simulink library "xbsDSP48_r3"  (Simulink 5.0)
libraries: xbsIndex_r3 x429, xbsDSP48_r3 x2
(part 3 of 8)

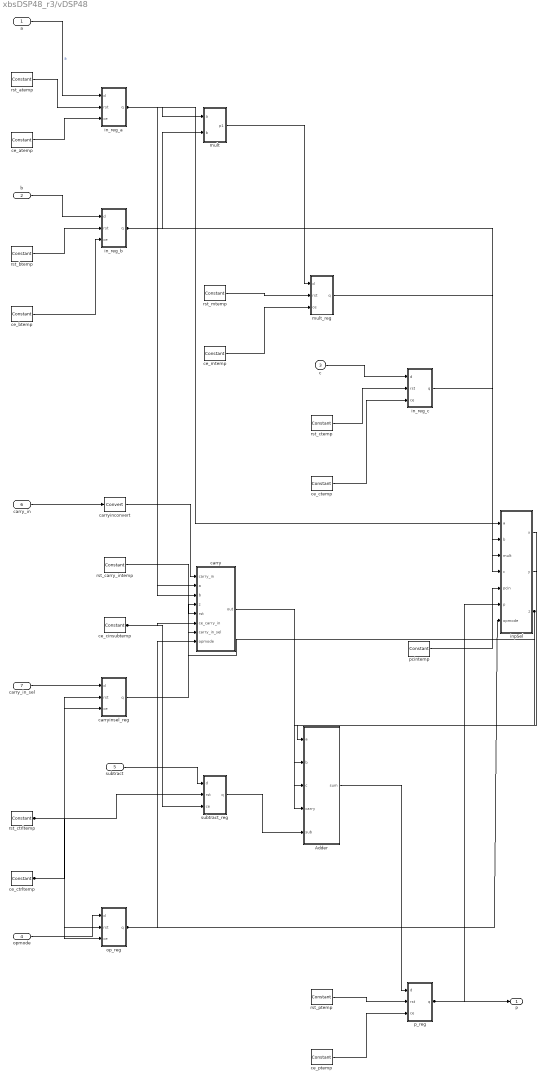
== system xbsDSP48_r3/vDSP48 ==
  a : Inport
  b : Inport  Port=2
  c : Inport  Port=3
  opmode : Inport  Port=4
  subtract : Inport  Port=5
  carry_in : Inport  Port=6
  carry_in_sel : Inport  Port=7
  Adder : Subsystem
  carry : Subsystem
  carryinconvert : xbsIndex_r3/Convert  arith_type=Unsigned  n_bits=1  bin_pt=0  quantization=Truncate  overflow=Wrap  latency=0  explicit_period=off  period=1  dbl_ovrd=off  show_param=off  inserted_by_tool=off  pipeline=off
      settings: xl_area=[0, 0, 0, 0, 0, 0, 0]
  carryinsel_reg : Subsystem  mask{nreg=pipeline_carryinsel, pnreg=1}
      mask prompts: nreg "Number of registers"; pnreg "Previous number of register"
      mask init: same as xbsDSP48_r3/DSP48reg
      mask Display:
      | patch([0 iWidth iWidth 0],[0 0 iHeight iHeight] , bg);
      | patch(logoX,logoY , fg);
      | text(iCx-6,iCy,'z');
      | text(iCx,iCy+4,str);
      | port_label('input',1,'d');
      | port_label('input',2,'rst');
      | port_label('input',3,'ce');
      | port_label('output',1,'q');
      | plot([0 0 iWidth iWidth 0], [0 iHeight iHeight 0 0]);
  ce_atemp : xbsIndex_r3/Constant  const=1  equ=P=C  arith_type=Boolean  n_bits=1  bin_pt=0  opselect=C  inp2=PCIN>>17  opr=+  inp1=P  carry=CIN  iostate=0  explicit_period=on  period=1  dbl_ovrd=off
  ce_btemp : xbsIndex_r3/Constant  const=1  equ=P=C  arith_type=Boolean  n_bits=1  bin_pt=0  opselect=C  inp2=PCIN>>17  opr=+  inp1=P  carry=CIN  iostate=0  explicit_period=on  period=1  dbl_ovrd=off
  ce_cinsubtemp : xbsIndex_r3/Constant  const=1  equ=P=C  arith_type=Boolean  n_bits=1  bin_pt=0  opselect=C  inp2=PCIN>>17  opr=+  inp1=P  carry=CIN  iostate=0  explicit_period=on  period=1  dbl_ovrd=off
  ce_ctemp : xbsIndex_r3/Constant  const=1  equ=P=C  arith_type=Boolean  n_bits=1  bin_pt=0  opselect=C  inp2=PCIN>>17  opr=+  inp1=P  carry=CIN  iostate=0  explicit_period=on  period=1  dbl_ovrd=off
  ce_ctrltemp : xbsIndex_r3/Constant  const=1  equ=P=C  arith_type=Boolean  n_bits=1  bin_pt=0  opselect=C  inp2=PCIN>>17  opr=+  inp1=P  carry=CIN  iostate=0  explicit_period=on  period=1  dbl_ovrd=off
  ce_mtemp : xbsIndex_r3/Constant  const=1  equ=P=C  arith_type=Boolean  n_bits=1  bin_pt=0  opselect=C  inp2=PCIN>>17  opr=+  inp1=P  carry=CIN  iostate=0  explicit_period=on  period=1  dbl_ovrd=off
  ce_ptemp : xbsIndex_r3/Constant  const=1  equ=P=C  arith_type=Boolean  n_bits=1  bin_pt=0  opselect=C  inp2=PCIN>>17  opr=+  inp1=P  carry=CIN  iostate=0  explicit_period=on  period=1  dbl_ovrd=off
  in_reg_a : Subsystem  mask{nreg=pipeline_a-1, pnreg=1}
      mask prompts: nreg "Number of registers"; pnreg "Previous number of register"
      mask init: same as xbsDSP48_r3/DSP48reg
      mask Display:
      | patch([0 iWidth iWidth 0],[0 0 iHeight iHeight] , bg);
      | patch(logoX,logoY , fg);
      | text(iCx-6,iCy,'z');
      | text(iCx,iCy+4,str);
      | port_label('input',1,'d');
      | port_label('input',2,'rst');
      | port_label('input',3,'ce');
      | port_label('output',1,'q');
      | plot([0 0 iWidth iWidth 0], [0 iHeight iHeight 0 0]);
  in_reg_b : Subsystem  mask{nreg=pipeline_b- 1, pnreg=1}
      mask prompts: nreg "Number of registers"; pnreg "Previous number of register"
      mask init: same as xbsDSP48_r3/DSP48reg
      mask Display:
      | patch([0 iWidth iWidth 0],[0 0 iHeight iHeight] , bg);
      | patch(logoX,logoY , fg);
      | text(iCx-6,iCy,'z');
      | text(iCx,iCy+4,str);
      | port_label('input',1,'d');
      | port_label('input',2,'rst');
      | port_label('input',3,'ce');
      | port_label('output',1,'q');
      | plot([0 0 iWidth iWidth 0], [0 iHeight iHeight 0 0]);
  in_reg_c : Subsystem  mask{nreg=pipeline_c, pnreg=1}
      mask prompts: nreg "Number of registers"; pnreg "Previous number of register"
      mask init: same as xbsDSP48_r3/DSP48reg
      mask Display:
      | patch([0 iWidth iWidth 0],[0 0 iHeight iHeight] , bg);
      | patch(logoX,logoY , fg);
      | text(iCx-6,iCy,'z');
      | text(iCx,iCy+4,str);
      | port_label('input',1,'d');
      | port_label('input',2,'rst');
      | port_label('input',3,'ce');
      | port_label('output',1,'q');
      | plot([0 0 iWidth iWidth 0], [0 iHeight iHeight 0 0]);
  inpSel : Subsystem
  mult : Subsystem
  mult_reg : Subsystem  mask{nreg=pipeline_mult, pnreg=1}
      mask prompts: nreg "Number of registers"; pnreg "Previous number of register"
      mask init: same as xbsDSP48_r3/DSP48reg
      mask Display:
      | patch([0 iWidth iWidth 0],[0 0 iHeight iHeight] , bg);
      | patch(logoX,logoY , fg);
      | text(iCx-6,iCy,'z');
      | text(iCx,iCy+4,str);
      | port_label('input',1,'d');
      | port_label('input',2,'rst');
      | port_label('input',3,'ce');
      | port_label('output',1,'q');
      | plot([0 0 iWidth iWidth 0], [0 iHeight iHeight 0 0]);
  op_reg : Subsystem  mask{nreg=pipeline_opmode, pnreg=1}
      mask prompts: nreg "Number of registers"; pnreg "Previous number of register"
      mask init: same as xbsDSP48_r3/DSP48reg
      mask Display:
      | patch([0 iWidth iWidth 0],[0 0 iHeight iHeight] , bg);
      | patch(logoX,logoY , fg);
      | text(iCx-6,iCy,'z');
      | text(iCx,iCy+4,str);
      | port_label('input',1,'d');
      | port_label('input',2,'rst');
      | port_label('input',3,'ce');
      | port_label('output',1,'q');
      | plot([0 0 iWidth iWidth 0], [0 iHeight iHeight 0 0]);
  p_reg : Subsystem  mask{nreg=pipeline_p, pnreg=1}
      mask prompts: nreg "Number of registers"; pnreg "Previous number of register"
      mask init: same as xbsDSP48_r3/DSP48reg
      mask Display:
      | patch([0 iWidth iWidth 0],[0 0 iHeight iHeight] , bg);
      | patch(logoX,logoY , fg);
      | text(iCx-6,iCy,'z');
      | text(iCx,iCy+4,str);
      | port_label('input',1,'d');
      | port_label('input',2,'rst');
      | port_label('input',3,'ce');
      | port_label('output',1,'q');
      | plot([0 0 iWidth iWidth 0], [0 iHeight iHeight 0 0]);
  pcintemp : xbsIndex_r3/Constant  const=1  equ=P=C  arith_type="Signed  (2's comp)"  n_bits=48  bin_pt=0  opselect=C  inp2=PCIN>>17  opr=+  inp1=P  carry=CIN  iostate=0  explicit_period=on  period=1  dbl_ovrd=off
  rst_atemp : xbsIndex_r3/Constant  const=0  equ=P=C  arith_type=Boolean  n_bits=1  bin_pt=0  opselect=C  inp2=PCIN>>17  opr=+  inp1=P  carry=CIN  iostate=0  explicit_period=on  period=1  dbl_ovrd=off
  rst_btemp : xbsIndex_r3/Constant  const=0  equ=P=C  arith_type=Boolean  n_bits=1  bin_pt=0  opselect=C  inp2=PCIN>>17  opr=+  inp1=P  carry=CIN  iostate=0  explicit_period=on  period=1  dbl_ovrd=off
  rst_carry_intemp : xbsIndex_r3/Constant  const=0  equ=P=C  arith_type=Boolean  n_bits=1  bin_pt=0  opselect=C  inp2=PCIN>>17  opr=+  inp1=P  carry=CIN  iostate=0  explicit_period=on  period=1  dbl_ovrd=off
  rst_ctemp : xbsIndex_r3/Constant  const=0  equ=P=C  arith_type=Boolean  n_bits=1  bin_pt=0  opselect=C  inp2=PCIN>>17  opr=+  inp1=P  carry=CIN  iostate=0  explicit_period=on  period=1  dbl_ovrd=off
  rst_ctrltemp : xbsIndex_r3/Constant  const=0  equ=P=C  arith_type=Boolean  n_bits=1  bin_pt=0  opselect=C  inp2=PCIN>>17  opr=+  inp1=P  carry=CIN  iostate=0  explicit_period=on  period=1  dbl_ovrd=off
  rst_mtemp : xbsIndex_r3/Constant  const=0  equ=P=C  arith_type=Boolean  n_bits=1  bin_pt=0  opselect=C  inp2=PCIN>>17  opr=+  inp1=P  carry=CIN  iostate=0  explicit_period=on  period=1  dbl_ovrd=off
  rst_ptemp : xbsIndex_r3/Constant  const=0  equ=P=C  arith_type=Boolean  n_bits=1  bin_pt=0  opselect=C  inp2=PCIN>>17  opr=+  inp1=P  carry=CIN  iostate=0  explicit_period=on  period=1  dbl_ovrd=off
  subtract_reg : Subsystem  mask{nreg=pipeline_sub, pnreg=1}
      mask prompts: nreg "Number of registers"; pnreg "Previous number of register"
      mask init: same as xbsDSP48_r3/DSP48reg
      mask Display:
      | patch([0 iWidth iWidth 0],[0 0 iHeight iHeight] , bg);
      | patch(logoX,logoY , fg);
      | text(iCx-6,iCy,'z');
      | text(iCx,iCy+4,str);
      | port_label('input',1,'d');
      | port_label('input',2,'rst');
      | port_label('input',3,'ce');
      | port_label('output',1,'q');
      | plot([0 0 iWidth iWidth 0], [0 iHeight iHeight 0 0]);
  P : Outport
  wires:
  in_reg_a/1(q) -> mult/1(a), carry/2(a), inpSel/1(a)
  inpSel/3(z) -> Adder/3(c), carry/4(z)
  op_reg/1(q) -> inpSel/7(opmode), carry/8(opmode)
  in_reg_b/1(q) -> mult/2(b), inpSel/2(b), carry/3(b)
  p_reg/1(q) -> P/1, inpSel/6(p)
  rst_ctrltemp/1 -> op_reg/2(rst), subtract_reg/2(rst), carryinsel_reg/2(rst)
  ce_ctrltemp/1 -> carryinsel_reg/3(ce), op_reg/3(ce)
  ce_cinsubtemp/1 -> carry/6(ce_carry_in), subtract_reg/3(ce)
  pcintemp/1 -> inpSel/5(pcin)
  b/1 -> in_reg_b/1(d)
  carry_in_sel/1 -> carryinsel_reg/1(d)
  carry_in/1 -> carryinconvert/1
  opmode/1 -> op_reg/1(d)
  a/1 -> in_reg_a/1(d)  "a"
  subtract/1 -> subtract_reg/1(d)
  c/1 -> in_reg_c/1(d)
  carryinconvert/1 -> carry/1(carry_in)
  in_reg_c/1(q) -> inpSel/4(c)
  mult/1(p1) -> mult_reg/1(d)
  mult_reg/1(q) -> inpSel/3(mult)
  inpSel/1(x) -> Adder/1(a)
  inpSel/2(y) -> Adder/2(b)
  Adder/1(sum) -> p_reg/1(d)
  subtract_reg/1(q) -> Adder/5(sub)
  carry/1(out) -> Adder/4(carry)
  carryinsel_reg/1(q) -> carry/7(carry_in_sel)
  rst_atemp/1 -> in_reg_a/2(rst)
  rst_btemp/1 -> in_reg_b/2(rst)
  rst_ctemp/1 -> in_reg_c/2(rst)
  rst_ptemp/1 -> p_reg/2(rst)
  rst_mtemp/1 -> mult_reg/2(rst)
  rst_carry_intemp/1 -> carry/5(rst)
  ce_atemp/1 -> in_reg_a/3(ce)
  ce_btemp/1 -> in_reg_b/3(ce)
  ce_ctemp/1 -> in_reg_c/3(ce)
  ce_ptemp/1 -> p_reg/3(ce)
  ce_mtemp/1 -> mult_reg/3(ce)

== system xbsDSP48_r3/vMultTemplate ==
  In1 : Inport
  In2 : Inport  Port=2
  In3 : Inport  Port=3
  In4 : Inport  Port=4
  In5 : Inport  Port=5
  In6 : Inport  Port=6
  In7 : Inport  Port=7
  AlignP : xbsIndex_r3/Reinterpret  force_arith_type=on  arith_type=Unsigned  force_bin_pt=on  bin_pt=0  force_valid=on
  ConvertP : xbsIndex_r3/Convert  arith_type="Signed  (2's comp)"  n_bits=48  bin_pt=0  quantization=Truncate  overflow=Wrap  latency=0  explicit_period=off  period=1  dbl_ovrd=off  show_param=off  inserted_by_tool=off  pipeline=off
      settings: xl_area=[0, 0, 0, 0, 0, 0, 0]
  DSP48 : Subsystem  mask(Xilinx vDSP48){pipeline_a=1, use_b=Direct from B port, pipeline_b=1, pipeline_bcin=0, pipeline_c=on, pipeline_p=on, pipeline_mult=on, pipeline_opmode=on, pipeline_sub=on, pipeline_carryin=on, pipeline_carryinsel=on, use_creg=on, use_pcin=off, use_pcout=off, use_bcout=off, access_rst=on, rst_all=off, rst_a=off, rst_b=off, rst_c=off, rst_p=off, rst_mult=off, rst_carry_in=off, rst_ctrl=off, access_en=on, en_all=off, en_a=off, en_b=off, en_c=off, en_p=off, en_mult=off, en_carry_in=off, en_ctrl=off, period=2, statestr=|1|Direct from B port|1|0|on|on|on|on|on|on|on|on|off|off|off|on|off|off|off|off|off|off|off|off|on|off|off|off|off|off|off|off|off|2}
      mask prompts: pipeline_a "Pipeline Input A"; use_b "B Input"; pipeline_b "Pipeline Input B"; pipeline_bcin "Pipeline Input BCIN"; pipeline_c "Pipeline Input C"; pipeline_p "Pipeline P"; pipeline_mult "Pipeline Multiplier"; pipeline_opmode "Pipeline Opmode"; pipeline_sub "Pipeline Subtract"; pipeline_carryin "Pipeline Carry In"; pipeline_carryinsel "Pipeline Carry In Sel"; use_creg "Provide C port"; use_pcin "Provide PCIN port"; use_pcout "Provide PCOUT port"; use_bcout "Provide BCOUT"; access_rst "---------------------------Access Reset Port Control------------------------------------"; rst_all "Provide Global Reset Port"; rst_a "Provide Reset Port for A"; rst_b "Provide Reset Port for B"; rst_c "Provide Reset Port for C"; rst_p "Provide Reset Port for P"; rst_mult "Provide Reset Port for Multiplier"; rst_carry_in "Provide Reset Port for Carry In"; rst_ctrl "Provide Reset Port for Controls (Subtract, CarryInSel, OpMode)"; access_en "----------------------------Access Enable Port Control---------------------------------"; en_all "Provide Global Enable Port"; en_a "Provide Enable for Port A"; en_b "Provide Enable for Port B"; en_c "Provide Enable for Port C"; en_p "Provide Enable for Port P"; en_mult "Provide Enable for Multiplier"; en_carry_in "Provide Enable for Carry In"; en_ctrl "Provide Enable Port for Controls (Subtract, CarryInSel, OpMode)"; period "Sample Period"
      mask init:
      | this_gcb = gcb;
      | set_param(this_gcb,'linkstatus','none');
      | xlgenvDSP48callback(this_gcb);
      mask StyleString: popup(0|1|2),popup(Direct from B port|Cascaded from BCIN port),popup(0|1|2),popup(0|1|2),checkbox,checkbox,checkbox,checkbox,checkbox,checkbox,checkbox,checkbox,checkbox,checkbox,checkbox,checkbox,checkbox,checkbox,checkbox,checkbox,checkbox,checkbox,checkbox,checkbox,checkbox,checkbox,checkbox,checkbox,checkbox,checkbox,checkbox,checkbox,checkbox,edit,edit
  UDType : xbsIndex_r3/Convert  arith_type="Signed  (2's comp)"  n_bits=48  bin_pt=0  quantization=Truncate  overflow=Wrap  latency=0  explicit_period=off  period=1  dbl_ovrd=off  show_param=off  inserted_by_tool=off  pipeline=off
      settings: xl_area=[0, 0, 0, 0, 0, 0, 0]
  Out1 : Outport
  wires:
  DSP48/1(P) -> ConvertP/1
  ConvertP/1 -> AlignP/1
  AlignP/1 -> UDType/1
  In1/1 -> DSP48/1(a)
  In7/1 -> DSP48/2(b)
  UDType/1 -> Out1/1
  In3/1 -> DSP48/4(opmode)
  In4/1 -> DSP48/5(subtract)
  In6/1 -> DSP48/7(carry_in_sel)
  In5/1 -> DSP48/6(carry_in)
  In2/1 -> DSP48/3(c)

== system xbsDSP48_r3/vMultTemplatenc ==
  In1 : Inport
  In2 : Inport  Port=2
  In3 : Inport  Port=3
  In4 : Inport  Port=4
  In5 : Inport  Port=5
  In6 : Inport  Port=6
  In7 : Inport  Port=7
  AlignP : xbsIndex_r3/Reinterpret  force_arith_type=on  arith_type=Unsigned  force_bin_pt=on  bin_pt=0  force_valid=on
  ConvertP : xbsIndex_r3/Convert  arith_type="Signed  (2's comp)"  n_bits=48  bin_pt=0  quantization=Truncate  overflow=Wrap  latency=0  explicit_period=off  period=1  dbl_ovrd=off  show_param=off  inserted_by_tool=off  pipeline=off
      settings: xl_area=[0, 0, 0, 0, 0, 0, 0]
  DSP48 : Subsystem  mask(Xilinx vDSP48){pipeline_a=1, use_b=Direct from B port, pipeline_b=1, pipeline_bcin=0, pipeline_c=on, pipeline_p=on, pipeline_mult=on, pipeline_opmode=on, pipeline_sub=on, pipeline_carryin=on, pipeline_carryinsel=on, use_creg=off, use_pcin=off, use_pcout=off, use_bcout=off, access_rst=on, rst_all=off, rst_a=off, rst_b=off, rst_c=off, rst_p=off, rst_mult=off, rst_carry_in=off, rst_ctrl=off, access_en=on, en_all=off, en_a=off, en_b=off, en_c=off, en_p=off, en_mult=off, en_carry_in=off, en_ctrl=off, period=1, statestr=|1|Direct from B port|1|0|on|on|on|on|on|on|on|off|off|off|off|on|off|off|off|off|off|off|off|off|on|off|off|off|off|off|off|off|off|1}
      mask prompts: pipeline_a "Pipeline Input A"; use_b "B Input"; pipeline_b "Pipeline Input B"; pipeline_bcin "Pipeline Input BCIN"; pipeline_c "Pipeline Input C"; pipeline_p "Pipeline P"; pipeline_mult "Pipeline Multiplier"; pipeline_opmode "Pipeline Opmode"; pipeline_sub "Pipeline Subtract"; pipeline_carryin "Pipeline Carry In"; pipeline_carryinsel "Pipeline Carry In Sel"; use_creg "Provide C port"; use_pcin "Provide PCIN port"; use_pcout "Provide PCOUT port"; use_bcout "Provide BCOUT"; access_rst "---------------------------Access Reset Port Control------------------------------------"; rst_all "Provide Global Reset Port"; rst_a "Provide Reset Port for A"; rst_b "Provide Reset Port for B"; rst_c "Provide Reset Port for C"; rst_p "Provide Reset Port for P"; rst_mult "Provide Reset Port for Multiplier"; rst_carry_in "Provide Reset Port for Carry In"; rst_ctrl "Provide Reset Port for Controls (Subtract, CarryInSel, OpMode)"; access_en "----------------------------Access Enable Port Control---------------------------------"; en_all "Provide Global Enable Port"; en_a "Provide Enable for Port A"; en_b "Provide Enable for Port B"; en_c "Provide Enable for Port C"; en_p "Provide Enable for Port P"; en_mult "Provide Enable for Multiplier"; en_carry_in "Provide Enable for Carry In"; en_ctrl "Provide Enable Port for Controls (Subtract, CarryInSel, OpMode)"; period "Sample Period"
      mask init:
      | this_gcb = gcb;
      | set_param(this_gcb,'linkstatus','none');
      | xlgenvDSP48callback(this_gcb);
      mask StyleString: popup(0|1|2),popup(Direct from B port|Cascaded from BCIN port),popup(0|1|2),popup(0|1|2),checkbox,checkbox,checkbox,checkbox,checkbox,checkbox,checkbox,checkbox,checkbox,checkbox,checkbox,checkbox,checkbox,checkbox,checkbox,checkbox,checkbox,checkbox,checkbox,checkbox,checkbox,checkbox,checkbox,checkbox,checkbox,checkbox,checkbox,checkbox,checkbox,edit,edit
  Terminator : Terminator
  UDType : xbsIndex_r3/Convert  arith_type="Signed  (2's comp)"  n_bits=48  bin_pt=0  quantization=Truncate  overflow=Wrap  latency=0  explicit_period=off  period=1  dbl_ovrd=off  show_param=off  inserted_by_tool=off  pipeline=off
      settings: xl_area=[0, 0, 0, 0, 0, 0, 0]
  Out1 : Outport
  wires:
  DSP48/1(P) -> ConvertP/1
  ConvertP/1 -> AlignP/1
  AlignP/1 -> UDType/1
  In1/1 -> DSP48/1(a)
  In7/1 -> DSP48/2(b)
  UDType/1 -> Out1/1
  In3/1 -> DSP48/3(opmode)
  In4/1 -> DSP48/4(subtract)
  In6/1 -> DSP48/6(carry_in_sel)
  In5/1 -> DSP48/5(carry_in)
  In2/1 -> Terminator/1

== system xbsDSP48_r3/DSP48 Macro/Aligncoeff ==
  In1 : Inport
  Align : xbsIndex_r3/Convert  arith_type="Signed  (2's comp)"  n_bits=n_bits  bin_pt=bin_pt  quantization=Truncate  overflow=Wrap  latency=0  explicit_period=off  period=1  dbl_ovrd=off  show_param=off  inserted_by_tool=off  pipeline=off
      settings: xl_area=[0, 0, 0, 0, 0, 0, 0]
  Prec : xbsIndex_r3/Convert  arith_type="Signed  (2's comp)"  n_bits=portwidth  bin_pt=0  quantization=Truncate  overflow=Wrap  latency=0  explicit_period=off  period=1  dbl_ovrd=off  show_param=off  inserted_by_tool=off  pipeline=off
      settings: xl_area=[0, 0, 0, 0, 0, 0, 0]
  Reinterpret : xbsIndex_r3/Reinterpret  force_arith_type=off  arith_type=Unsigned  force_bin_pt=on  bin_pt=0  force_valid=on
  Out1 : Outport
  wires:
  Prec/1 -> Out1/1
  In1/1 -> Align/1
  Reinterpret/1 -> Prec/1
  Align/1 -> Reinterpret/1

== system xbsDSP48_r3/DSP48 Macro/AlignnoneC ==
  In1 : Inport
  Align : xbsIndex_r3/Convert  arith_type="Signed  (2's comp)"  n_bits=n_bits  bin_pt=bin_pt  quantization=Truncate  overflow=Wrap  latency=0  explicit_period=off  period=1  dbl_ovrd=off  show_param=off  inserted_by_tool=off  pipeline=off
      settings: xl_area=[0, 0, 0, 0, 0, 0, 0]
  Prec : xbsIndex_r3/Convert  arith_type="Signed  (2's comp)"  n_bits=portwidth  bin_pt=0  quantization=Truncate  overflow=Wrap  latency=0  explicit_period=off  period=1  dbl_ovrd=off  show_param=off  inserted_by_tool=off  pipeline=off
      settings: xl_area=[0, 0, 0, 0, 0, 0, 0]
  Reinterpret : xbsIndex_r3/Reinterpret  force_arith_type=off  arith_type=Unsigned  force_bin_pt=on  bin_pt=0  force_valid=on
  Out1 : Outport
  wires:
  Prec/1 -> Out1/1
  In1/1 -> Align/1
  Reinterpret/1 -> Prec/1
  Align/1 -> Reinterpret/1

== system xbsDSP48_r3/DSP48 Macro/C_reg ==
  d : Inport
  rst : Inport  Port=2
  ce : Inport  Port=3
  Register1 : xbsIndex_r3/Register  init=0  reg_only_valid=off  explicit_period=off  period=1  rst=on  en=on  out_en=off  dbl_ovrd=off  show_param=off
      settings: xl_area=[0, 0, 0, 0, 0, 0, 0]
  Register2 : xbsIndex_r3/Register  init=0  reg_only_valid=off  explicit_period=off  period=1  rst=on  en=on  out_en=off  dbl_ovrd=off  show_param=off
      settings: xl_area=[0, 0, 0, 0, 0, 0, 0]
  q : Outport
  wires:
  d/1 -> Register1/1
  rst/1 -> Register1/2, Register2/2
  ce/1 -> Register1/3, Register2/3
  Register1/1 -> Register2/1
  Register2/1 -> q/1

== system xbsDSP48_r3/DSP48 Macro/DSP48 ==
  In1 : Inport
  In2 : Inport  Port=2
  In3 : Inport  Port=3
  In4 : Inport  Port=4
  In5 : Inport  Port=5
  In6 : Inport  Port=6
  In7 : Inport  Port=7
  AlignP : xbsIndex_r3/Reinterpret  force_arith_type=on  arith_type=Unsigned  force_bin_pt=on  bin_pt=11  force_valid=on
  ConvertP : xbsIndex_r3/Convert  arith_type="Signed  (2's comp)"  n_bits=48  bin_pt=0  quantization=Truncate  overflow=Wrap  latency=0  explicit_period=off  period=1  dbl_ovrd=off  show_param=off  inserted_by_tool=off  pipeline=off
      settings: xl_area=[0, 0, 0, 0, 0, 0, 0]
  DSP48 : xbsIndex_r3/DSP48  pipeline_a=1  use_b=Cascaded from BCIN Port  pipeline_b=1  pipeline_bcin=1  pipeline_c=on  pipeline_p=on  pipeline_mult=on  pipeline_opmode=on  pipeline_sub=on  pipeline_carryin=on  pipeline_carryinsel=on  use_op=off  use_creg=on  use_pcin=off  use_pcout=off  use_bcout=off  access_rst=off  rst_all=off  rst_a=off  rst_b=off  rst_bcin=off  rst_c=off  rst_mult=off  rst_p=off  rst_ctrl=off  rst_carry_in=off  access_en=off  en_all=off  en_a=off  en_b=off  en_bcin=off  en_c=off  en_mult=off  en_p=off  en_carry_in=off  en_ctrl=off  explicit_period=on  period=1  dbl_ovrd=off
      settings: xl_area=[0, 0, 0, 0, 0, 0, 0]  xl_use_area=on
  UDType : xbsIndex_r3/Convert  arith_type="Signed  (2's comp)"  n_bits=16  bin_pt=2  quantization=Truncate  overflow=Wrap  latency=0  explicit_period=off  period=1  dbl_ovrd=off  show_param=off  inserted_by_tool=off  pipeline=off
      settings: xl_area=[0, 0, 0, 0, 0, 0, 0]
  Out1 : Outport
  wires:
  In7/1 -> DSP48/2
  In1/1 -> DSP48/1
  In2/1 -> DSP48/3
  In5/1 -> DSP48/6
  In6/1 -> DSP48/7
  In4/1 -> DSP48/5
  In3/1 -> DSP48/4
  UDType/1 -> Out1/1
  AlignP/1 -> UDType/1
  ConvertP/1 -> AlignP/1
  DSP48/1 -> ConvertP/1

== system xbsDSP48_r3/DSP48 Macro/reg_Subtract ==
  d : Inport
  rst : Inport  Port=2
  ce : Inport  Port=3
  Register1 : xbsIndex_r3/Register  init=0  reg_only_valid=off  explicit_period=off  period=1  rst=on  en=on  out_en=off  dbl_ovrd=off  show_param=off
      settings: xl_area=[0, 0, 0, 0, 0, 0, 0]
  Register2 : xbsIndex_r3/Register  init=0  reg_only_valid=off  explicit_period=off  period=1  rst=on  en=on  out_en=off  dbl_ovrd=off  show_param=off
      settings: xl_area=[0, 0, 0, 0, 0, 0, 0]
  q : Outport
  wires:
  d/1 -> Register1/1
  rst/1 -> Register1/2, Register2/2
  ce/1 -> Register1/3, Register2/3
  Register1/1 -> Register2/1
  Register2/1 -> q/1

== system xbsDSP48_r3/DSP48 Macro/reg_carry ==
  d : Inport
  rst : Inport  Port=2
  ce : Inport  Port=3
  Register1 : xbsIndex_r3/Register  init=0  reg_only_valid=off  explicit_period=off  period=1  rst=on  en=on  out_en=off  dbl_ovrd=off  show_param=off
      settings: xl_area=[0, 0, 0, 0, 0, 0, 0]
  Register2 : xbsIndex_r3/Register  init=0  reg_only_valid=off  explicit_period=off  period=1  rst=on  en=on  out_en=off  dbl_ovrd=off  show_param=off
      settings: xl_area=[0, 0, 0, 0, 0, 0, 0]
  q : Outport
  wires:
  d/1 -> Register1/1
  rst/1 -> Register1/2, Register2/2
  ce/1 -> Register1/3, Register2/3
  Register1/1 -> Register2/1
  Register2/1 -> q/1

== system xbsDSP48_r3/DSP48 Macro/reg_opmode ==
  d : Inport
  rst : Inport  Port=2
  ce : Inport  Port=3
  Register1 : xbsIndex_r3/Register  init=0  reg_only_valid=off  explicit_period=off  period=1  rst=on  en=on  out_en=off  dbl_ovrd=off  show_param=off
      settings: xl_area=[0, 0, 0, 0, 0, 0, 0]
  Register2 : xbsIndex_r3/Register  init=0  reg_only_valid=off  explicit_period=off  period=1  rst=on  en=on  out_en=off  dbl_ovrd=off  show_param=off
      settings: xl_area=[0, 0, 0, 0, 0, 0, 0]
  q : Outport
  wires:
  d/1 -> Register1/1
  rst/1 -> Register1/2, Register2/2
  ce/1 -> Register1/3, Register2/3
  Register1/1 -> Register2/1
  Register2/1 -> q/1

== system xbsDSP48_r3/DSP48_Adder/opmode ==
  opmode : xbsIndex_r3/Constant  const=35  equ=P=C  arith_type=Unsigned  n_bits=7  bin_pt=0  opselect=C  inp2=PCIN>>17  opr=+  inp1=P  carry=CIN  iostate=0  explicit_period=off  period=1  dbl_ovrd=off
  op : Outport
  wires:
  opmode/1 -> op/1

== system xbsDSP48_r3/DSP48_Mult/opmode ==
  opmode : xbsIndex_r3/Constant  const=5  equ=P=C  arith_type=Unsigned  n_bits=7  bin_pt=0  opselect=C  inp2=PCIN>>17  opr=+  inp1=P  carry=CIN  iostate=0  explicit_period=off  period=1  dbl_ovrd=off
  op : Outport
  wires:
  opmode/1 -> op/1
